simulink model "IM_Model"  (R2023a)
settings: Solver=VariableStepAuto  StartTime=0.0  StopTime=10.0  RelTol=1e-3
undefined symbols (not defined in the file): B, J, k, K_T, L_m, L_r, L_s, np, R_r, R_s, Tm, V_rd, V_rq, Vmax, w
settings Model: Creator=11048  LastModifiedBy=11048

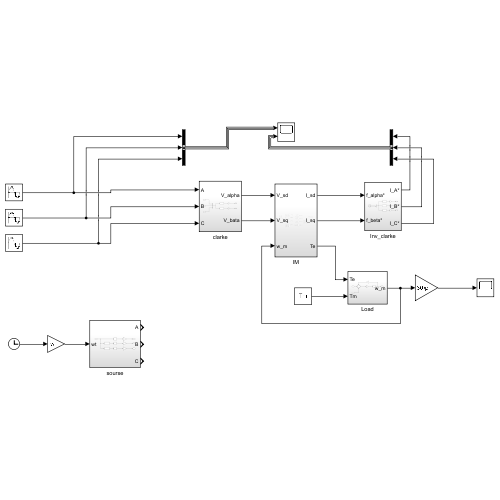
[thumbnail: Simulink's stored preview of the top-level diagram]
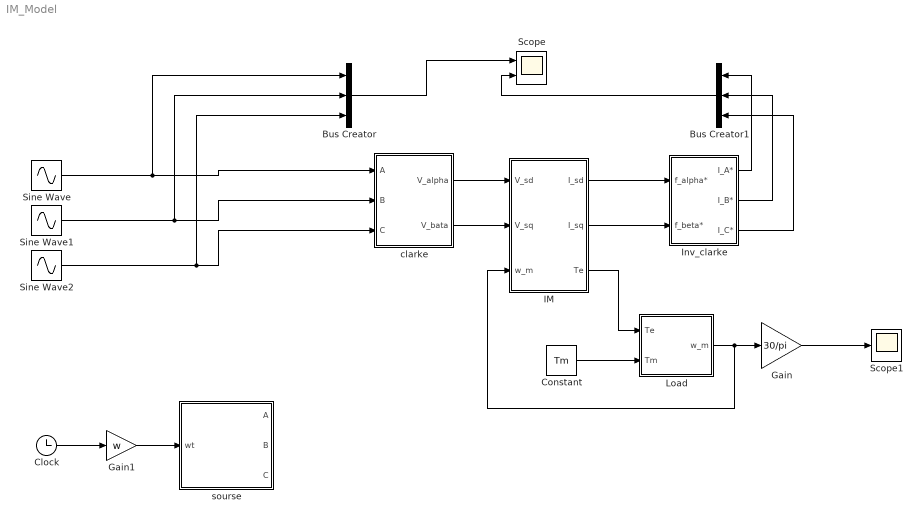
== system IM_Model ==
  Bus Creator : BusCreator  Inputs=3
  Bus Creator1 : BusCreator  Inputs=3
  Clock : Clock
  Constant : Constant  Value=Tm
  Gain : Gain  Gain=30/pi
  Gain1 : Gain  Gain=w
  IM : Subsystem
  Inv_clarke : Subsystem
  Load : Subsystem
  Scope : Scope  NumInputPorts=2
  Scope1 : Scope
  Sine Wave : Sin  Amplitude=220  Frequency=2*pi*50  SampleTime=0.00001
  Sine Wave1 : Sin  Amplitude=220  Frequency=2*pi*50  Phase=(-2/3)*pi  SampleTime=0.00001
  Sine Wave2 : Sin  Amplitude=220  Frequency=2*pi*50  Phase=(2/3)*pi  SampleTime=0.00001
  clarke : Subsystem
  sourse : Subsystem
  wires:
  Constant/1 -> Load/2(Tm)
  IM/3(Te) -> Load/1(Te)
  Load/1(w_m) -> IM/3(w_m), Gain/1
  clarke/1(V_alpha) -> IM/1(V_sd)
  clarke/2(V_bata) -> IM/2(V_sq)
  IM/1(I_sd) -> Inv_clarke/1(f_alpha*)
  IM/2(I_sq) -> Inv_clarke/2(f_beta*)
  Clock/1 -> Gain1/1
  Gain1/1 -> sourse/1(wt)
  Bus Creator/1 -> Scope/1
  Inv_clarke/1(I_A*) -> Bus Creator1/1
  Inv_clarke/2(I_B*) -> Bus Creator1/2
  Inv_clarke/3(I_C*) -> Bus Creator1/3
  Bus Creator1/1 -> Scope/2
  Gain/1 -> Scope1/1
  Sine Wave/1 -> Bus Creator/1, clarke/1(A)
  Sine Wave1/1 -> Bus Creator/2, clarke/2(B)
  Sine Wave2/1 -> Bus Creator/3, clarke/3(C)

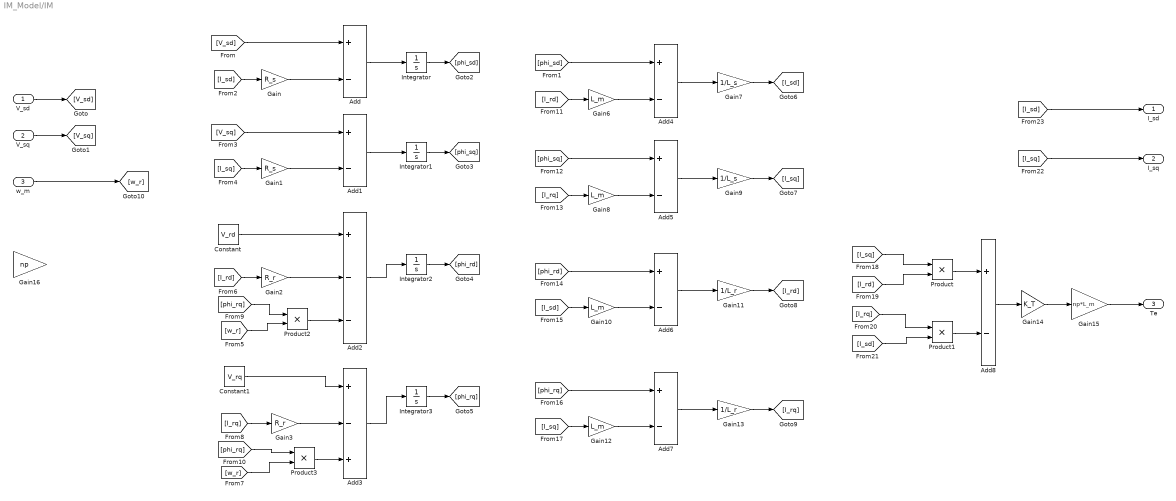
== system IM_Model/IM ==
  V_sd : Inport
  V_sq : Inport  Port=2
  w_m : Inport  Port=3
  Add{,1,4..8} (7 alike) : Sum  Inputs=+-
  Add2 : Sum  Inputs=+--
  Add3 : Sum  Inputs=+-+
  Constant : Constant  Value=V_rd
  Constant1 : Constant  Value=V_rq
  Gain : Gain  Gain=R_s
  Gain1 : Gain  Gain=R_s
  Gain{6,8,10,12} (4 alike) : Gain  Gain=L_m
  Gain11 : Gain  Gain=1/L_r
  Gain13 : Gain  Gain=1/L_r
  Gain14 : Gain  Gain=K_T
  Gain15 : Gain  Gain=np*L_m
  Gain16 : Gain  Gain=np
  Gain2 : Gain  Gain=R_r
  Gain3 : Gain  Gain=R_r
  Gain7 : Gain  Gain=1/L_s
  Gain9 : Gain  Gain=1/L_s
  Integrator{,1..3} (4 alike) : Integrator
  Product{,1..3} (4 alike) : Product
  I_sd : Outport
  I_sq : Outport  Port=2
  Te : Outport  Port=3
  wires:
  Gain8/1 -> Add5/2
  Add/1 -> Integrator/1
  [V_sq] -> Add1/1
  [I_rq] -> Product1/1
  [V_sd] -> Add/1
  V_sd/1 -> [V_sd]
  Integrator1/1 -> [phi_sq]
  Integrator/1 -> [phi_sd]
  Gain11/1 -> [I_rd]
  [I_sq] -> Gain12/1
  Add5/1 -> Gain9/1
  [I_rd] -> Product/2
  [phi_sd] -> Add4/1
  [I_sq] -> Product/1
  Integrator3/1 -> [phi_rq]
  Product/1 -> Add8/1
  Gain15/1 -> Te/1
  [I_rd] -> Gain2/1
  Constant1/1 -> Add3/1
  [phi_sq] -> Add5/1
  [I_sq] -> I_sq/1
  Add7/1 -> Gain13/1
  [I_rq] -> Gain8/1
  Add8/1 -> Gain14/1
  [I_sd] -> Gain10/1
  Product1/1 -> Add8/2
  [I_rd] -> Gain6/1
  Constant/1 -> Add2/1
  Gain7/1 -> [I_sd]
  [I_sd] -> Gain/1
  Gain13/1 -> [I_rq]
  [I_sd] -> I_sd/1
  Add1/1 -> Integrator1/1
  Add4/1 -> Gain7/1
  [I_sq] -> Gain1/1
  Gain1/1 -> Add1/2
  Add2/1 -> Integrator2/1
  Gain/1 -> Add/2
  Integrator2/1 -> [phi_rd]
  Gain2/1 -> Add2/2
  Gain14/1 -> Gain15/1
  [phi_rd] -> Add6/1
  Add6/1 -> Gain11/1
  Gain10/1 -> Add6/2
  Gain3/1 -> Add3/2
  [I_sd] -> Product1/2
  V_sq/1 -> [V_sq]
  [phi_rq] -> Add7/1
  Gain9/1 -> [I_sq]
  Add3/1 -> Integrator3/1
  Gain12/1 -> Add7/2
  [I_rq] -> Gain3/1
  Gain6/1 -> Add4/2
  [w_r] -> Product2/2
  [phi_rq] -> Product2/1
  Product2/1 -> Add2/3
  [w_r] -> Product3/2
  [phi_rq] -> Product3/1
  Product3/1 -> Add3/3
  w_m/1 -> [w_r]

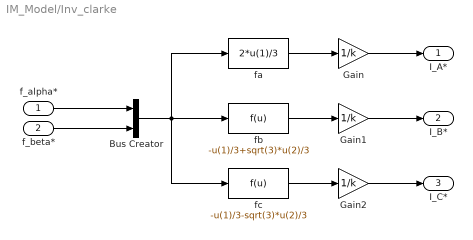
== system IM_Model/Inv_clarke ==
  f_alpha* : Inport
  f_beta* : Inport  Port=2
  Bus Creator : BusCreator  Inputs=2
  Gain : Gain  Gain=1/k
  Gain1 : Gain  Gain=1/k
  Gain2 : Gain  Gain=1/k
  fa : Fcn  Expr=2*u(1)/3
  fb : Fcn  Expr=-u(1)/3+sqrt(3)*u(2)/3
  fc : Fcn  Expr=-u(1)/3-sqrt(3)*u(2)/3
  I_A* : Outport
  I_B* : Outport  Port=2
  I_C* : Outport  Port=3
  wires:
  Bus Creator/1 -> fc/1, fb/1, fa/1
  f_alpha*/1 -> Bus Creator/1
  f_beta*/1 -> Bus Creator/2
  fa/1 -> Gain/1
  Gain/1 -> I_A*/1
  fb/1 -> Gain1/1
  Gain1/1 -> I_B*/1
  fc/1 -> Gain2/1
  Gain2/1 -> I_C*/1

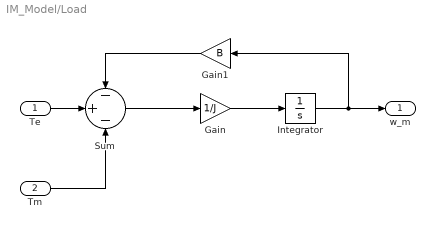
== system IM_Model/Load ==
  Te : Inport
  Tm : Inport  Port=2
  Gain : Gain  Gain=1/J
  Gain1 : Gain  Gain=B
  Integrator : Integrator
  Sum : Sum  Inputs=-+-
  w_m : Outport
  wires:
  Integrator/1 -> Gain1/1, w_m/1
  Sum/1 -> Gain/1
  Gain/1 -> Integrator/1
  Tm/1 -> Sum/3
  Te/1 -> Sum/2
  Gain1/1 -> Sum/1

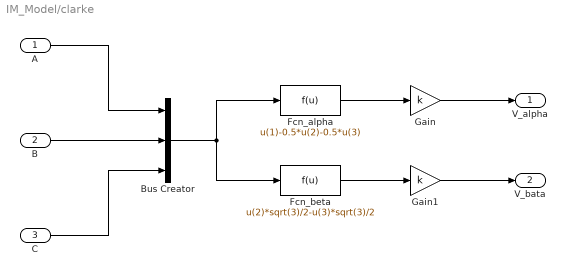
== system IM_Model/clarke ==
  A : Inport
  B : Inport  Port=2
  C : Inport  Port=3
  Bus Creator : BusCreator  Inputs=3
  Fcn_alpha : Fcn  Expr=u(1)-0.5*u(2)-0.5*u(3)
  Fcn_beta : Fcn  Expr=u(2)*sqrt(3)/2-u(3)*sqrt(3)/2
  Gain : Gain  Gain=k
  Gain1 : Gain  Gain=k
  V_alpha : Outport
  V_bata : Outport  Port=2
  wires:
  Bus Creator/1 -> Fcn_beta/1, Fcn_alpha/1
  A/1 -> Bus Creator/1
  C/1 -> Bus Creator/3
  B/1 -> Bus Creator/2
  Fcn_alpha/1 -> Gain/1
  Gain/1 -> V_alpha/1
  Fcn_beta/1 -> Gain1/1
  Gain1/1 -> V_bata/1

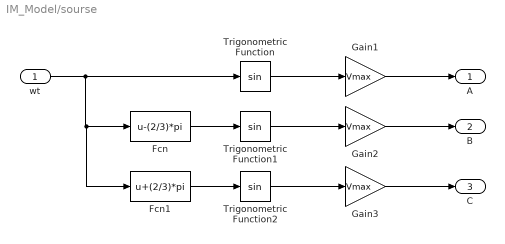
== system IM_Model/sourse ==
  wt : Inport
  Fcn : Fcn  Expr=u-(2/3)*pi
  Fcn1 : Fcn  Expr=u+(2/3)*pi
  Gain1 : Gain  Gain=Vmax
  Gain2 : Gain  Gain=Vmax
  Gain3 : Gain  Gain=Vmax
  Trigonometric Function : Trigonometry
  Trigonometric Function1 : Trigonometry
  Trigonometric Function2 : Trigonometry
  A : Outport
  B : Outport  Port=2
  C : Outport  Port=3
  wires:
  Trigonometric Function/1 -> Gain1/1
  wt/1 -> Fcn1/1, Fcn/1, Trigonometric Function/1
  Fcn/1 -> Trigonometric Function1/1
  Fcn1/1 -> Trigonometric Function2/1
  Gain3/1 -> C/1
  Gain1/1 -> A/1
  Gain2/1 -> B/1
  Trigonometric Function2/1 -> Gain3/1
  Trigonometric Function1/1 -> Gain2/1
